simulink model "Reaching"  (R2021b)
settings: Solver=FixedStepDiscrete  StartTime=0.0  StopTime=inf  FixedStep=0.001  RelTol=1e-3
libraries: PhanTorque_3Dof_Library_64Bits x1, vrlib x1
settings Model: Creator=carlos.aldana  LastModifiedBy=manti
settings SolverCC: AlgebraicLoopSolver=TrustRegion
settings DataIOCC: LimitDataPoints=on  SaveFormat=Array  ReturnWorkspaceOutputs=off
settings OptimizationCC: BlockReduction=off  BooleanDataType=off  LifeSpan=inf
settings DebuggingCC: SaveWithParameterizedLinksMsg=none  UnderspecifiedInitializationDetection=Classic  MergeDetectMultiDrivingBlocksExec=none  SignalResolutionControl=TryResolveAllWithWarning  AllowSymbolicDim=off  SFUnexpectedBacktrackingDiag=warning  SFNoUnconditionalDefaultTransitionDiag=warning  SFExecutionAtInitializationDiag=none  SFMachineParentedDataDiag=warning  ArithmeticOperatorsInVariantConditions=warning
settings HardwareCC: ProdBitPerPointer=32  ProdBitPerSizeT=32  ProdBitPerPtrDiffT=32  ProdLargestAtomicFloat=None  ProdIntDivRoundTo=Undefined  ProdEndianess=Unspecified  ProdWordSize=32  ProdHWDeviceType=32-bit Generic  TargetUnknown=on
settings ModelReferenceCC: PropagateSignalLabelsOutOfModel=off
settings SFSimCC: SimUseLocalCustomCode=off  CustomCodeUndefinedFunction=UseInterfaceOnly
settings RTWCC: RTWUseLocalCustomCode=off
settings CodeAppCC: StateflowObjectComments=on
settings GRTTargetCC: TargetLangStandard=C89/C90 (ANSI)
settings ConfigComp: CovMetricSettings=dw  CovSaveCumulativeToWorkspaceVar=on  CovSaveSingleToWorkspaceVar=on  CovExternalEMLEnable=off  CovSFcnEnable=off

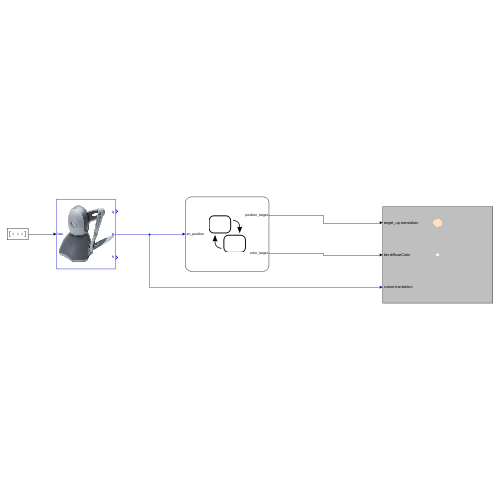
[thumbnail: Simulink's stored preview of the top-level diagram]
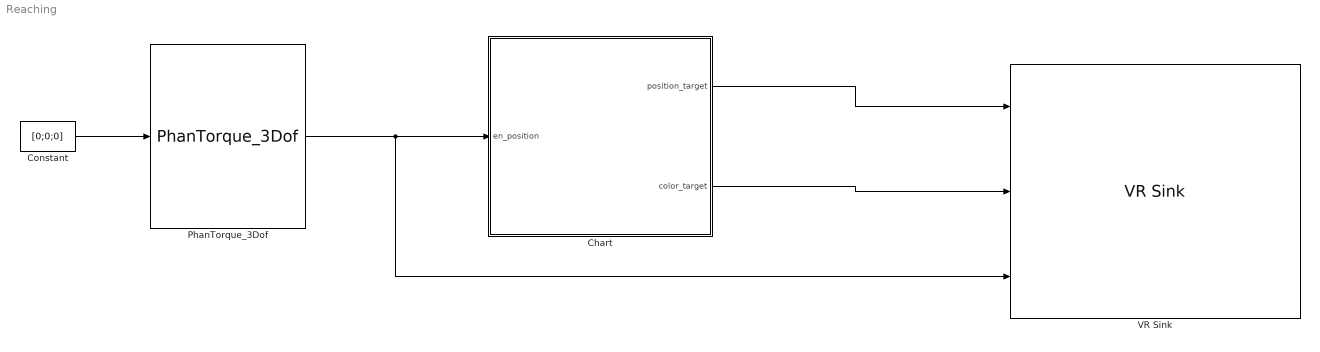
== system Reaching ==
  Chart : Stateflow chart  TreatAsAtomicUnit=on
  Constant : Constant  Value=[0;0;0]
  PhanTorque_3Dof : PhanTorque_3Dof_Library_64Bits/PhanTorque_3Dof  Haptic_Name='Default Device'
  VR Sink : vrlib/VR Sink  InstantiateOnLoad=on  SampleTime=0.1  ViewEnable=on  RemoteChange=off  RemoteView=off  FieldsWritten=target_up.translation.3.1.1.double#ber.diffuseColor.3.1.1.double#cursor.translation.3.1.1.double  WorldFileName=8_palline_color.wrl  AutoView=off  VideoDimensions=[]  AllowVariableSize=off  FigureProperties="{'Position', 'Name', 'Viewpoint', 'CameraBound', 'CameraDirection', 'CameraPosition', 'CameraUpVector', 'ZoomFactor', 'Antialiasing', 'Headlight', 'Lighting', 'NavPanel', 'Sound', 'StatusBar', 'Stereo3D', 'Stereo3DCameraOffset', 'Stereo3DHIT', 'ToolBar', 'Textures', 'Transparency', 'Triad', 'Wireframe', 'NavZones', 'NavMode', 'NavSpeed', 'CaptureFileFormat', 'CaptureFileName', 'Record2DCompressMethod', 'Record2DCompressQuality', 'Record2D', 'Record2DFileName', 'Record2DFPS'; [5.0000000000000000e+00   9.2000000000000000e+01   5.7600000000000000e+02   3.5000000000000000e+02], '', '_untitled_1', 'on', [0.0000000000000000e+00   0.0000000000000000e+00  -1.0000000000000000e+00], [0.0000000000000000e+00   0.0000000000000000e+00   0.0000000000000000e+00], [0.0000000000000000e+00   1.0000000000000000e+00   0.0000000000000000e+00], [1.0000000000000000e+00], 'on', 'on', 'on', 'halfbar', 'on', 'on', 'off', [1.0000000149011612e-01], [0.0000000000000000e+00], 'on', 'on', 'on', 'none', 'off', 'off', 'fly', 'normal', 'tif', '%f_anim_%n.tif', 'auto', [7.5000000000000000e+01], 'off', '%f_anim_%n.avi', 'auto'}"
  wires:
  Constant/1 -> PhanTorque_3Dof/1
  PhanTorque_3Dof/2 -> VR Sink/3, Chart/1(en_position)
  Chart/1(position_target) -> VR Sink/1
  Chart/2(color_target) -> VR Sink/2

== stateflow chart Reaching/Chart ==
  state Inizializing
    entry:
    radious=0.1;
    threshold=0.01;
    color_target=[1 0 0];
    counter=1;
  state Inizializing2
    entry:
    angle=2*pi*rand;
  state Finish
  state New_target
    entry:
    position_target=[radious*cos(angle); radious*sin(angle); 0]
    d1=(en_position(1,1)-position_target(1,1))^2+((en_position(2,1)-position_target(2,1))^2);
    d=sqrt(d1);
    during:
    d1=(en_position(1,1)-position_target(1,1))^2+((en_position(2,1)-position_target(2,1))^2);
    d=sqrt(d1);
    %dx=en_position-position_target(1,1); %distance
    %dy=en_position-position_target(2,1);
  state changecolor1
    color_target=[0 0 1];
    during:
    d1=(en_position(1,1)-position_target(1,1))^2+((en_position(2,1)-position_target(2,1))^2);
    d=sqrt(d1);
  state hometarget_on
    position_target = [0; 0 ;0];
    color_target=[0 0 1];
    during:
    d1=(en_position(1,1)-position_target(1,1))^2+((en_position(2,1)-position_target(2,1))^2);
    d=sqrt(d1);
  state changecolor2
    color_target=[1 0 1];
    during:
    d1=(en_position(1,1)-position_target(1,1))^2+((en_position(2,1)-position_target(2,1))^2);
    d=sqrt(d1);
  (default) -> Inizializing
  Inizializing2 -> Finish [order 2] : [counter>=10]
  Inizializing -> Inizializing2
  changecolor2 -> Inizializing2 : [after(2,sec) && d<threshold]
  Inizializing2 -> New_target [order 1] : [counter<10]
  changecolor1 -> New_target [order 2] : [d>threshold]
  New_target -> changecolor1 : [d<threshold]
  hometarget_on -> changecolor1 [order 2] : [d>threshold]
  changecolor1 -> hometarget_on [order 1] : [after(1,sec) && d<threshold]{counter=counter+1;}
  hometarget_on -> changecolor2 [order 1] : [d<threshold]
  data: position_target output; color_target output; en_position input; counter local; d local; radious local; angle local; threshold local; d1 local
